simulink model "Subsystem"  (R2016a)
settings: Solver=VariableStepAuto  StartTime=0.0  StopTime=120  RelTol=1e-3
values from neighbouring files (symbols this model uses):
  b = 50.0    [Data_Dic.sldd]    (also in MAT_FILE.mat = 50)
  m = 1000.0    [Data_Dic.sldd]    (also in MAT_FILE.mat = 1000)
settings Model: DataDictionary=Data_Dic.sldd  Creator=Admin  LastModifiedBy=Admin
settings DataIOCC: SaveOutput=off  SaveTime=off

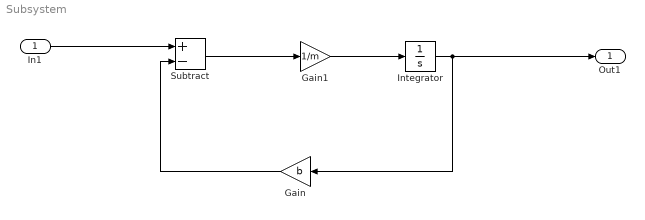
== system Subsystem ==
  In1 : Inport  OutDataTypeStr=double  PortDimensions=1  SampleTime=0
  Gain : Gain  Gain=b
  Gain1 : Gain  Gain=1/m
  Integrator : Integrator
  Subtract : Sum  Inputs=+-
  Out1 : Outport  OutDataTypeStr=double  PortDimensions=1  SampleTime=0
  wires:
  Subtract/1 -> Gain1/1
  Gain1/1 -> Integrator/1
  Integrator/1 -> Gain/1, Out1/1
  In1/1 -> Subtract/1
  Gain/1 -> Subtract/2
